simulink model "LPF_model"  (R2018a)
settings: Solver=FixedStepDiscrete  StartTime=0.0  StopTime=30  FixedStep=0.01  RelTol=1e-3  EnableMultiTasking=on
PreLoadFcn:
  | pass=1;
settings Model: Creator=lenovo  LastModifiedBy=lenovo
settings DataIOCC: LimitDataPoints=on  SaveFormat=Array
settings OptimizationCC: LifeSpan=1
settings DebuggingCC: SolverPrmCheckMsg=warning  SFUnexpectedBacktrackingDiag=warning  SFNoUnconditionalDefaultTransitionDiag=warning  SFExecutionAtInitializationDiag=none
settings HardwareCC: ProdBitPerInt=16  ProdBitPerPointer=8  ProdBitPerSizeT=16  ProdBitPerPtrDiffT=16  ProdLargestAtomicFloat=None  ProdEndianess=Unspecified  ProdWordSize=8  ProdShiftRightIntArith=off  ProdHWDeviceType=Intel->8051 Compatible
settings ModelReferenceCC: PropagateSignalLabelsOutOfModel=off
settings SFSimCC: MATLABDynamicMemAlloc=off
settings RTWCC: SystemTargetFile=ert.tlc  GenCodeOnly=on  TemplateMakefile=ert_default_tmf  GenerateReport=on  IncludeHyperlinkInReport=on  LaunchReport=on
settings CodeAppCC: IgnoreCustomStorageClasses=off  StateflowObjectComments=on
settings ERTTargetCC: MultiwordLength=2048  SupportContinuousTime=on  ERTCustomFileTemplate=example_file_process.tlc  ConvertIfToSwitch=off  SuppressUnreachableDefaultCases=off
settings ConfigComp: CovMetricSettings=dw  CovHtmlReporting=on  CovSaveCumulativeToWorkspaceVar=on  CovSaveSingleToWorkspaceVar=on  CovExternalEMLEnable=off  CovSFcnEnable=off

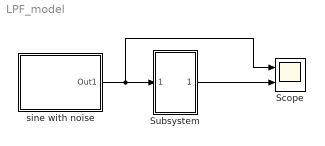
== system LPF_model ==
  Scope : Scope  NumInputPorts=2
  Subsystem : Subsystem
  sine with noise : Subsystem
      mask Display:
      | t=0:0.01:10;
      | noise=normrnd(0,0.5,[1,length(t)]);
      | sin_with_noise=5*sin(t)+noise;
      | plot(t,sin_with_noise);
  wires:
  sine with noise/1(Out1) -> Subsystem/1(In1), Scope/1
  Subsystem/1(Out1) -> Scope/2

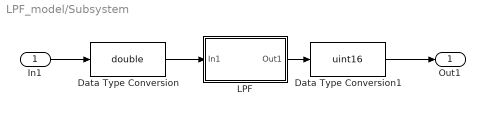
== system LPF_model/Subsystem ==
  In1 : Inport  OutDataTypeStr=uint16
  Data Type Conversion : DataTypeConversion  OutDataTypeStr=double
  Data Type Conversion1 : DataTypeConversion  OutDataTypeStr=uint16
  LPF : Subsystem
      mask Display:
      | num=1;
      | den=[1,1];
      | ts=tf(num,den);
      | P=bodeoptions;
      | P.PhaseVisible='off';
      | [mag,~,w]=bode(ts,P);
      | w=reshape(w,1,length(w));
      | mag=reshape(mag,1,length(w));
      | dB=20*log10(mag);
      | w=log10(w);
      | plot(w,dB);
  Out1 : Outport  OutDataTypeStr=uint16
  wires:
  In1/1 -> Data Type Conversion/1
  LPF/1(Out1) -> Data Type Conversion1/1
  Data Type Conversion1/1 -> Out1/1
  Data Type Conversion/1 -> LPF/1(In1)

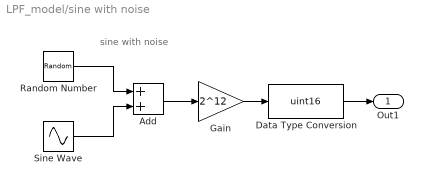
== system LPF_model/sine with noise ==
  note: sine with noise
  Add : Sum
  Data Type Conversion : DataTypeConversion  OutDataTypeStr=uint16  LockScale=on
  Gain : Gain  Gain=2^12
  Random Number : RandomNumber  Variance=0.5
  Sine Wave : Sin  Amplitude=5  Bias=8
  Out1 : Outport
  wires:
  Add/1 -> Gain/1
  Random Number/1 -> Add/1
  Sine Wave/1 -> Add/2
  Data Type Conversion/1 -> Out1/1
  Gain/1 -> Data Type Conversion/1

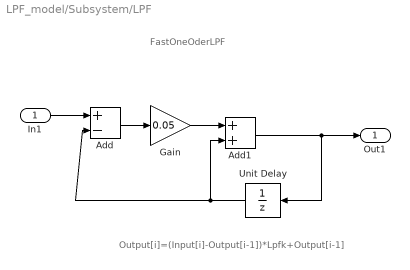
== system LPF_model/Subsystem/LPF ==
  note: Output[i]=(Input[i]-Output[i-1])*Lpfk+Output[i-1]
  note: FastOneOderLPF
  In1 : Inport
  Add : Sum  Inputs=+-
  Add1 : Sum
  Gain : Gain  Gain=0.05
  Unit Delay : UnitDelay  SampleTime=-1
  Out1 : Outport
  wires:
  In1/1 -> Add/1
  Add/1 -> Gain/1
  Gain/1 -> Add1/1
  Add1/1 -> Unit Delay/1, Out1/1
  Unit Delay/1 -> Add1/2, Add/2
